simulink model "power_switch"  (Simulink 6.0)
settings: Solver=ode15s  SolverMode=SingleTasking  StartTime=0.0  StopTime=0.2  RelTol=1e-3  AbsTol=1e-3
libraries: powerlib x11, powerlib_extras x1
settings Model: Creator=patrice  LastModifiedBy=batserve  ExtModeTrigMode=oneshot  ExtModeArmWhenConnect=off  ExtModeAutoUpdateStatusClock=off
settings SolverCC: MaxOrder=4
settings DataIOCC: LimitDataPoints=off  SignalLoggingName=sigsOut
settings OptimizationCC: BlockReduction=off  BooleanDataType=off
settings DebuggingCC: SolverPrmCheckMsg=none
settings HardwareCC: TargetUnknown=on
settings RTWCC: TemplateMakefile=grt_unix.tmf

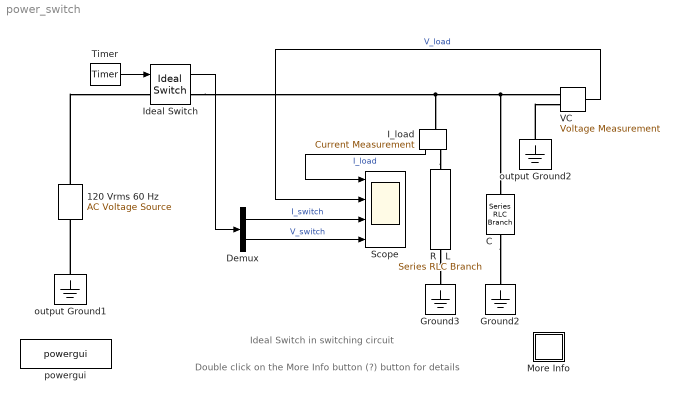
== system power_switch ==
  note: Double click on the More Info button (?) button for details
  note: Ideal Switch in switching circuit
  120 Vrms 60 Hz : powerlib/Electrical Sources/AC Voltage Source  Description=source block  Orientation=up  Amplitude=120*sqrt(2)  Phase=0  Frequency=60  SampleTime=0  Measurements=None
      settings: AttributesFormatString=\n
  C : powerlib/Elements/Series RLC Branch  Orientation=down  PhysicalDomain=powersysdomain  SubClassName=unknown  PortType=p1  LConnTagsString=__new0  RConnTagsString=__new0  Resistance=0  Inductance=0  Capacitance=10e-6  Measurements=None
  Demux : Demux  Outputs=2
  Ground2 : powerlib/Elements/Ground  Orientation=down  PhysicalDomain=powersysdomain  SubClassName=unknown  PortType=p1  LConnTagsString=a
  Ground3 : powerlib/Elements/Ground  Orientation=down  PhysicalDomain=powersysdomain  SubClassName=unknown  PortType=p1  LConnTagsString=a
  I_load : powerlib/Measurements/Current Measurement  Tag=PoWeRsYsTeMmEaSuReMeNt  Orientation=down  PhasorSimulation=off  OutputType=Magnitude  PSBequivalent=0
  Ideal Switch : powerlib/Power Electronics/Ideal Switch  Ron=0.01  Lon=1e-9  IC=1  Rs=inf  Cs=0.1e-6  Measurements=on
      settings: AttributesFormatString=\n
  More Info : Subsystem
      mask Display: disp('?')
  R   L : powerlib/Elements/Series RLC Branch  Orientation=down  PhysicalDomain=powersysdomain  SubClassName=unknown  PortType=p1  LConnTagsString=__new0  RConnTagsString=__new0  Resistance=10  Inductance=.1  Capacitance=inf  Measurements=None
  Scope : Scope  NumInputPorts=4
      settings: TimeRange=0.2  YMin=-20~-1500~-10.2014~-2000  YMax=15~1500~10.1871~2000  DataFormat=Array
  Timer : powerlib_extras/Control  Blocks/Timer  t="[0 3/60  8.25/60 ]"  e=[1 0 1]
  VC : powerlib/Measurements/Voltage Measurement  Tag=PoWeRsYsTeMmEaSuReMeNt  PhasorSimulation=off  OutputType=Magnitude  PSBequivalent=0
  output Ground1 : powerlib/Elements/Ground  Orientation=down  PhysicalDomain=powersysdomain  SubClassName=unknown  PortType=p1  LConnTagsString=a
  output Ground2 : powerlib/Elements/Ground  Orientation=down  PhysicalDomain=powersysdomain  SubClassName=unknown  PortType=p1  LConnTagsString=a
  powergui : powerlib/powergui  Priority=2  Frange=logspace(0,3,50)  Ylog=off  Xlog=off  save=off  variable=ZData  ZoomFFT=on  StartTime=0.0  cycles=1  DisplayStyle=off  fundamental=60  FreqAxis=off  MaxFrequency=1000  frequencyindice=1  frequencyindicesteady=1  RmsSteady=1  display=off  Ts=0  methode=off  frequency=60  echomessages=off
  wires:
  Demux/1 -> Scope/3  "I_switch"
  Demux/2 -> Scope/4  "V_switch"
  Timer/1 -> Ideal Switch/1
  Ideal Switch/1 -> Demux/1
  I_load/1 -> Scope/1  "I_load"
  VC/1 -> Scope/2  "V_load"
  connections:
  120 Vrms 60 Hz/RConn1 -- Ideal Switch/LConn1
  output Ground1/LConn1 -- 120 Vrms 60 Hz/LConn1
  R   L/RConn1 -- Ground3/LConn1
  C/RConn1 -- Ground2/LConn1
  output Ground2/LConn1 -- VC/LConn2
  I_load/RConn1 -- R   L/LConn1
  Ideal Switch/RConn1 -- I_load/LConn1 -- C/LConn1 -- VC/LConn1

== system power_switch/More Info ==
  note: The Ideal Switch is used to switch an RLC load on a 120V rms, 60 Hz voltage source.
      | The switch is initially closed.
      | It is turned off at t = 3 cycles (50 ms), then it is reclosed at t = 8.25 cycles (138 ms).
  note: This example illustrates the use of the Ideal Switch
      | ____________________________________________
  note: Observe that current chopping produces a load overvoltage at switch opening.
      | Also observe high switch curent spike when the capacitive circuit is re-energized at maximum source voltage.
